simulink model "ComponentTF"  (Simulink 7.5)
settings: Solver=ode45  StartTime=0.0  StopTime=inf  RelTol=1e-3
InitFcn:
  | a=1.25;
  | wn=2;
  | zeta=.5;
settings Model: Creator=dmanegol  LastModifiedBy=dmanegol

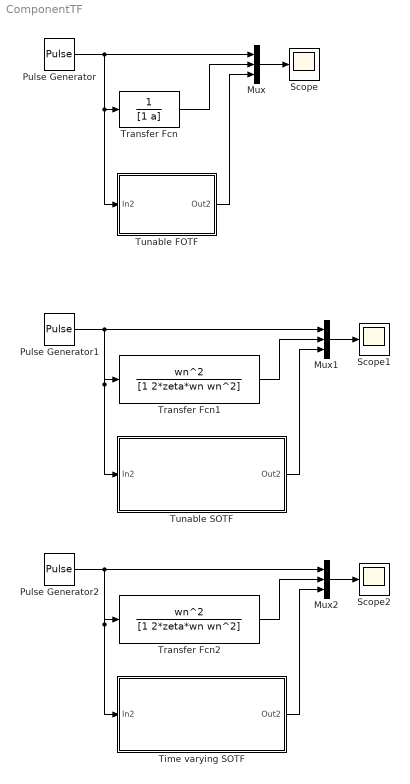
== system ComponentTF ==
  Mux : Mux  Inputs=3
  Mux1 : Mux  Inputs=3
  Mux2 : Mux  Inputs=3
  Pulse Generator : DiscretePulseGenerator  PulseType=Time based  Amplitude=1  Period=10  PulseWidth=50  PhaseDelay=0  SampleTime=1
  Pulse Generator1 : DiscretePulseGenerator  PulseType=Time based  Amplitude=1  Period=10  PulseWidth=50  PhaseDelay=0  SampleTime=1
  Pulse Generator2 : DiscretePulseGenerator  PulseType=Time based  Amplitude=1  Period=10  PulseWidth=50  PhaseDelay=0  SampleTime=1
  Scope : Scope
      settings: YMin=0  YMax=1
  Scope1 : Scope
      settings: YMin=-0.2  YMax=1.2
  Scope2 : Scope
      settings: TimeRange=10  YMin=-3  YMax=3  SaveName=ScopeData2
  Time varying SOTF : Subsystem
      mask Display: disp(strvcat(['Time varying natural'],['frequency (wn) and'],['damping (zeta)']))
  Transfer Fcn : TransferFcn  Denominator=[1 a]
  Transfer Fcn1 : TransferFcn  Numerator=wn^2  Denominator=[1 2*zeta*wn wn^2]
  Transfer Fcn2 : TransferFcn  Numerator=wn^2  Denominator=[1 2*zeta*wn wn^2]
  Tunable FOTF : Subsystem  mask{a=2}
      mask Display: disp(strvcat(['  1'],['------'],['s + a']))
  Tunable SOTF : Subsystem  mask{wn=2, zeta=.5}
      mask Display: disp(strvcat(['        wn^2'],['---------------------------------'],['s^2 + 2*zeta*wn*s + wn^2']))
  wires:
  Pulse Generator/1 -> Mux/1, Transfer Fcn/1, Tunable FOTF/1(In2)
  Transfer Fcn/1 -> Mux/2
  Tunable FOTF/1(Out2) -> Mux/3
  Mux/1 -> Scope/1
  Pulse Generator1/1 -> Tunable SOTF/1(In2), Transfer Fcn1/1, Mux1/1
  Transfer Fcn1/1 -> Mux1/2
  Tunable SOTF/1(Out2) -> Mux1/3
  Mux1/1 -> Scope1/1
  Pulse Generator2/1 -> Mux2/1, Transfer Fcn2/1, Time varying SOTF/1(In2)
  Transfer Fcn2/1 -> Mux2/2
  Time varying SOTF/1(Out2) -> Mux2/3
  Mux2/1 -> Scope2/1

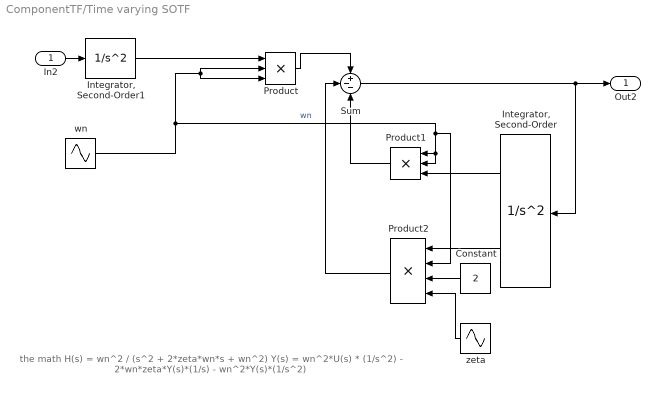
== system ComponentTF/Time varying SOTF ==
  note: the math
      | H(s) = wn^2 /  (s^2 + 2*zeta*wn*s + wn^2)
      | Y(s) = wn^2*U(s) * (1/s^2) - 2*wn*zeta*Y(s)*(1/s) - wn^2*Y(s)*(1/s^2)
  In2 : Inport
  Constant : Constant  Value=2
  "Integrator, Second-Order" : SecondOrderIntegrator
  "Integrator, Second-Order1" : SecondOrderIntegrator  ShowOutput=x
  Product : Product  Inputs=3  RndMeth=Zero
  Product1 : Product  Inputs=3  RndMeth=Zero
  Product2 : Product  Inputs=4  RndMeth=Zero
  Sum : Sum  Inputs=+--
  wn : Sin  Amplitude=5  Bias=7  Frequency=2e-4  Phase=0  Samples=10  SampleTime=0  Offset=0
  zeta : Sin  Amplitude=.25  Bias=.8  Frequency=1e-3  Phase=0  Samples=10  SampleTime=0  Offset=0
  Out2 : Outport
  wires:
  Product/1 -> Sum/1
  "Integrator, Second-Order1"/1 -> Product/1
  In2/1 -> "Integrator, Second-Order1"/1
  Product1/1 -> Sum/3
  Product2/1 -> Sum/2
  "Integrator, Second-Order"/2 -> Product2/1
  "Integrator, Second-Order"/1 -> Product1/3
  Sum/1 -> "Integrator, Second-Order"/1, Out2/1
  Constant/1 -> Product2/3
  zeta/1 -> Product2/4
  wn/1 -> Product/2, Product/3, Product1/1, Product1/2, Product2/2  "wn"

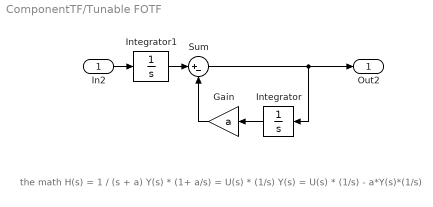
== system ComponentTF/Tunable FOTF ==
  note: the math
      | H(s) = 1 /  (s + a)
      | Y(s) * (1+ a/s) = U(s) * (1/s)
      | Y(s) = U(s) * (1/s) - a*Y(s)*(1/s)
  In2 : Inport
  Gain : Gain  Gain=a
  Integrator : Integrator
  Integrator1 : Integrator
  Sum : Sum  Inputs=|+-
  Out2 : Outport
  wires:
  Integrator/1 -> Gain/1
  Gain/1 -> Sum/2
  In2/1 -> Integrator1/1
  Sum/1 -> Integrator/1, Out2/1
  Integrator1/1 -> Sum/1

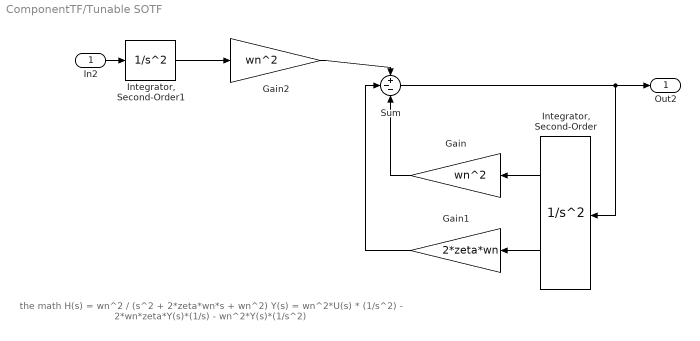
== system ComponentTF/Tunable SOTF ==
  note: the math
      | H(s) = wn^2 /  (s^2 + 2*zeta*wn*s + wn^2)
      | Y(s) = wn^2*U(s) * (1/s^2) - 2*wn*zeta*Y(s)*(1/s) - wn^2*Y(s)*(1/s^2)
  In2 : Inport
  Gain : Gain  Gain=wn^2
  Gain1 : Gain  Gain=2*zeta*wn
  Gain2 : Gain  Gain=wn^2
  "Integrator, Second-Order" : SecondOrderIntegrator
  "Integrator, Second-Order1" : SecondOrderIntegrator  ShowOutput=x
  Sum : Sum  Inputs=+--
  Out2 : Outport
  wires:
  Sum/1 -> Out2/1, "Integrator, Second-Order"/1
  "Integrator, Second-Order"/1 -> Gain/1
  "Integrator, Second-Order"/2 -> Gain1/1
  Gain1/1 -> Sum/2
  Gain/1 -> Sum/3
  In2/1 -> "Integrator, Second-Order1"/1
  "Integrator, Second-Order1"/1 -> Gain2/1
  Gain2/1 -> Sum/1
